simulink model "compassGaitSim_impacts"  (R2013a)
settings: Solver=ode45  StartTime=0.0  StopTime=20.0  FixedStep=0.01  MaxStep=0.02  MinStep=1e-8  RelTol=1e-3
values from neighbouring files (symbols this model uses):
  g = 9.81    [runSim.m]
  I1 = Is(1)    [PartialSolZeroDyn.m]    (also in impactDynamics_broken.m; runSim.m = 1)
  I2 = Is(2)    [PartialSolZeroDyn.m]    (also in impactDynamics_broken.m; runSim.m = 0.6)
  l1 = ls(1)    [PartialSolZeroDyn.m]    (also in impactDynamics_broken.m; runSim.m = 0.5)
  l2 = ls(2)    [PartialSolZeroDyn.m]    (also in impactDynamics_broken.m; runSim.m = 0.5)
  m1 = ms(1)    [PartialSolZeroDyn.m]    (also in impactDynamics_broken.m; runSim.m = 1.2)
  m2 = ms(2)    [PartialSolZeroDyn.m]    (also in impactDynamics_broken.m; runSim.m = 1.2)
  points = get(handles.uitable1, 'Data')'    [BezGui.m]    (also in BezGuiAttempt.m = [P0'; P1'; P2'; P3']; runSim.m = BezGuiAttempt')
undefined symbols (not defined in the file or in its folder): t1_0, t1d_0, t2_0, t2d_0
libraries: simulink x1
settings Model: CovHTMLOptions=-sRT=1 -aTS=1 -bRG=1 -bTC=1 -hTR=0 -nFC=0 -scm=1 -bcm=1 -xEv=0  Creator=yak  LastModifiedBy=yak

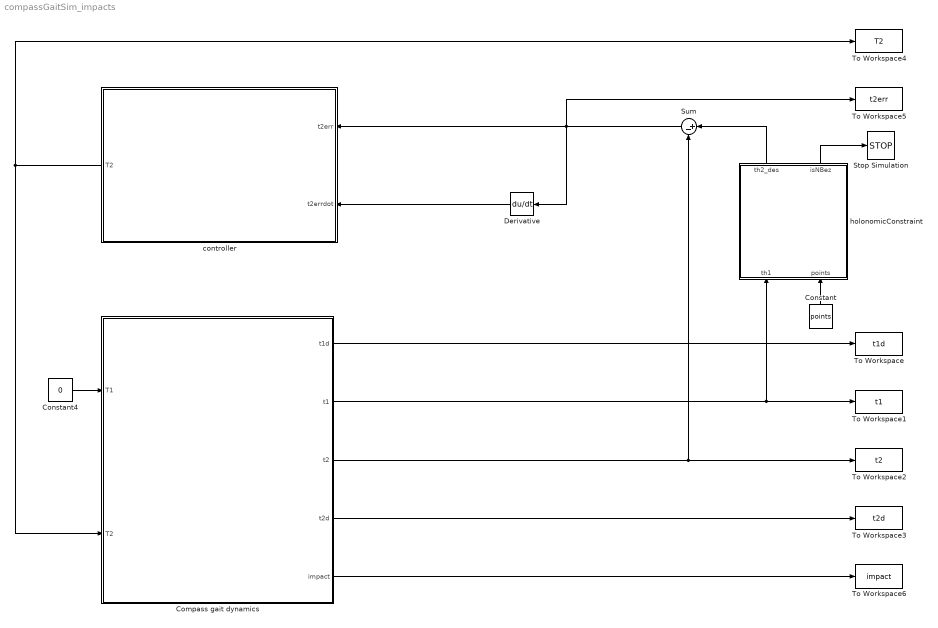
== system compassGaitSim_impacts ==
  Compass gait dynamics : Subsystem
  Constant : Constant  Value=points
  Constant4 : Constant  Value=0
  Derivative : Derivative
  Stop Simulation : Stop
  Sum : Sum  Inputs=|+-
  To Workspace : ToWorkspace  VariableName=t1d  SampleTime=-1  SaveFormat=Timeseries
  To Workspace1 : ToWorkspace  VariableName=t1  SampleTime=-1  SaveFormat=Timeseries
  To Workspace2 : ToWorkspace  VariableName=t2  SampleTime=-1  SaveFormat=Timeseries
  To Workspace3 : ToWorkspace  VariableName=t2d  SampleTime=-1  SaveFormat=Timeseries
  To Workspace4 : ToWorkspace  VariableName=T2  SampleTime=-1  SaveFormat=Timeseries
  To Workspace5 : ToWorkspace  VariableName=t2err  SampleTime=-1  SaveFormat=Timeseries
  To Workspace6 : ToWorkspace  VariableName=impact  SampleTime=-1  SaveFormat=Timeseries
  controller : MATLAB Function  TreatAsAtomicUnit=on
  holonomicConstraint : MATLAB Function  TreatAsAtomicUnit=on
  wires:
  controller/1(T2) -> Compass gait dynamics/2(T2), To Workspace4/1
  Compass gait dynamics/1(t1d) -> To Workspace/1
  Compass gait dynamics/2(t1) -> To Workspace1/1, holonomicConstraint/1(th1)
  Compass gait dynamics/3(t2) -> Sum/2, To Workspace2/1
  Compass gait dynamics/4(t2d) -> To Workspace3/1
  Constant4/1 -> Compass gait dynamics/1(T1)
  holonomicConstraint/1(th2_des) -> Sum/1
  Sum/1 -> To Workspace5/1, Derivative/1, controller/1(t2err)
  Derivative/1 -> controller/2(t2errdot)
  Constant/1 -> holonomicConstraint/2(points)
  holonomicConstraint/2(isNBez) -> Stop Simulation/1
  Compass gait dynamics/5(impact) -> To Workspace6/1

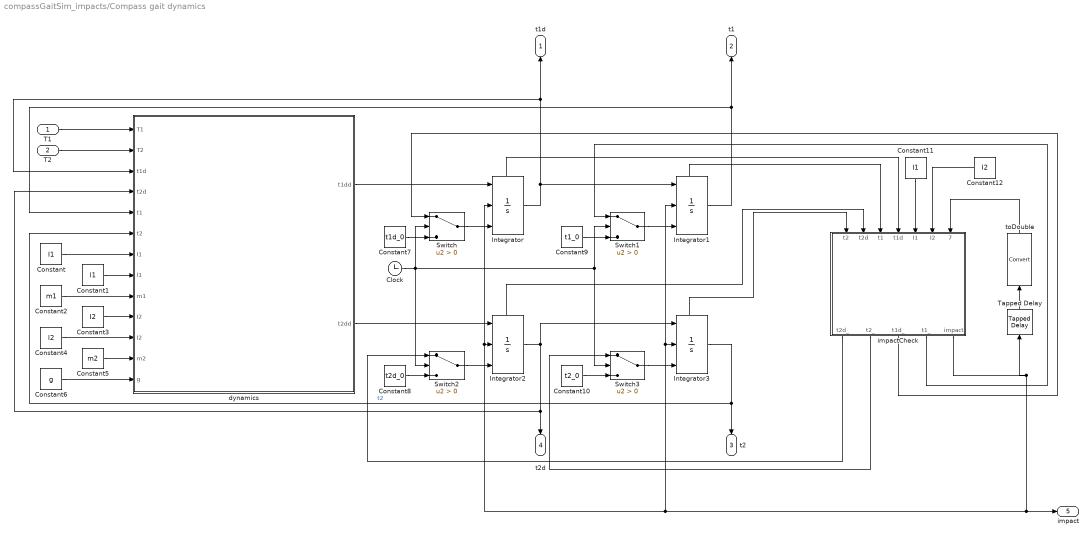
== system compassGaitSim_impacts/Compass gait dynamics ==
  T1 : Inport
  T2 : Inport  Port=2
  Clock : Clock
  Constant : Constant  Value=I1
  Constant1 : Constant  Value=l1
  Constant10 : Constant  Value=t2_0
  Constant11 : Constant  Value=I1
  Constant12 : Constant  Value=I2
  Constant2 : Constant  Value=m1
  Constant3 : Constant  Value=I2
  Constant4 : Constant  Value=l2
  Constant5 : Constant  Value=m2
  Constant6 : Constant  Value=g
  Constant7 : Constant  Value=t1d_0
  Constant8 : Constant  Value=t2d_0
  Constant9 : Constant  Value=t1_0
  Integrator{,1..3} (4 alike) : Integrator  ExternalReset=rising  InitialConditionSource=external  ShowStatePort=on
  Switch{,1..3} (4 alike) : Switch  Criteria=u2 > Threshold
  Tapped Delay : simulink/Discrete/Tapped Delay  vinit=1  samptime=-1  NumDelays=10  DelayOrder=Oldest  includeCurrent=off
  dynamics : MATLAB Function  TreatAsAtomicUnit=on
  impactCheck : MATLAB Function  TreatAsAtomicUnit=on
  toDouble : DataTypeConversion
  t1d : Outport
  t1 : Outport  Port=2
  t2 : Outport  Port=3
  t2d : Outport  Port=4
  impact : Outport  Port=5
  wires:
  T1/1 -> dynamics/1(T1)
  T2/1 -> dynamics/2(T2)
  dynamics/1(t1dd) -> Integrator/1
  Integrator/1 -> Integrator1/1, t1d/1, dynamics/3(t1d)
  Integrator2/1 -> Integrator3/1, t2d/1, dynamics/4(t2d)
  Integrator3/1 -> t2/1, dynamics/6(t2)  "t2"
  Integrator1/1 -> dynamics/5(t1), t1/1
  Constant2/1 -> dynamics/9(m1)
  Constant/1 -> dynamics/7(I1)
  Constant1/1 -> dynamics/8(l1)
  Constant3/1 -> dynamics/10(I2)
  Constant4/1 -> dynamics/11(l2)
  Constant5/1 -> dynamics/12(m2)
  Constant6/1 -> dynamics/13(g)
  Switch/1 -> Integrator/3
  Constant7/1 -> Switch/3
  Switch1/1 -> Integrator1/3
  Constant9/1 -> Switch1/3
  Switch2/1 -> Integrator2/3
  dynamics/2(t2dd) -> Integrator2/1
  Switch3/1 -> Integrator3/3
  Clock/1 -> Switch2/2, Switch3/2, Switch1/2, Switch/2
  Tapped Delay/1 -> toDouble/1
  impactCheck/5(impact) -> impact/1, Integrator1/2, Integrator3/2, Integrator/2, Integrator2/2, Tapped Delay/1
  toDouble/1 -> impactCheck/7(prev_impact)
  Integrator3/State -> impactCheck/1(t2)
  Integrator2/State -> impactCheck/2(t2d)
  Constant8/1 -> Switch2/3
  Constant10/1 -> Switch3/3
  impactCheck/1(t2d_) -> Switch2/1
  impactCheck/2(t2_) -> Switch3/1
  Integrator/State -> impactCheck/4(t1d)
  Integrator1/State -> impactCheck/3(t1)
  impactCheck/4(t1_) -> Switch1/1
  impactCheck/3(t1d_) -> Switch/1
  Constant11/1 -> impactCheck/5(I1)
  Constant12/1 -> impactCheck/6(I2)

== matlab function compassGaitSim_impacts/controller ==
  data: t2err input; t2errdot input; T2 output
function T2 = controller(t2err, t2errdot)
%#codegen

% Simple PD controller:
K_p = 1000;
K_d = 10;

t2err = mod(t2err, 2*pi);   % Ensure error is within 1 rotation

% Ensure error is in the range [-pi pi]
if t2err > pi
    t2err = -(2*pi - t2err);
elseif t2err < -pi
    t2err = 2*pi - t2err;
end

T2 = K_p*t2err + K_d*t2errdot;


end

== matlab function compassGaitSim_impacts/Compass gait dynamics/dynamics ==
  data: T1 input; t1dd output; T2 input; t1d input; t2d input; t1 input; t2 input; t2dd output; I1 input; l1 input; m1 input; I2 input; l2 input; m2 input; g input
function [t1dd, t2dd] = compassGaitDynamics(T1, T2, t1d, t2d, t1, t2, ...
    I1, l1, m1, I2, l2, m2, g)
%#codegen

c1 = cos(t1);
c2 = cos(t2);
s2 = sin(t2);
c12 = cos(t1 + t2);


% Equations in terms of T1 and T2 are derived, then the solution in terms
% of the angle accelerations have been pre-solved. The output is below.
t1dd = (4*I2*T1 - 4*I2*T2 + T1*l2^2*m2 - T2*l2^2*m2 - ...
    c1*g*l1*l2^2*m2^2 - 2*I2*c1*g*l1*m1 - 4*I2*c1*g*l1*m2 - ...
    2*T2*c2*l1*l2*m2 + (l1*l2^3*m2^2*s2*t1d^2)/2 + ...
    (l1*l2^3*m2^2*s2*t2d^2)/2 + 2*I2*l1*l2*m2*s2*t1d^2 + ...
    2*I2*l1*l2*m2*s2*t2d^2 - (c1*g*l1*l2^2*m1*m2)/2 + ...
    c2*l1^2*l2^2*m2^2*s2*t1d^2 + c2*c12*g*l1*l2^2*m2^2 + ...
    l1*l2^3*m2^2*s2*t1d*t2d + 4*I2*l1*l2*m2*s2*t1d*t2d)/ ...
    (- c2^2*l1^2*l2^2*m2^2 + l1^2*l2^2*m2^2 + ...
    4*I2*l1^2*m2 + I1*l2^2*m2 + 4*I1*I2);

t2dd = -(4*I2*T1 - 4*I1*T2 - 4*I2*T2 + T1*l2^2*m2 - 4*T2*l1^2*m2 - ...
    T2*l2^2*m2 - c1*g*l1*l2^2*m2^2 + 2*c12*g*l1^2*l2*m2^2 - ...
    2*I2*c1*g*l1*m1 - 4*I2*c1*g*l1*m2 + 2*I1*c12*g*l2*m2 + ...
    2*T1*c2*l1*l2*m2 - 4*T2*c2*l1*l2*m2 + (l1*l2^3*m2^2*s2*t1d^2)/2 + ...
    2*l1^3*l2*m2^2*s2*t1d^2 + (l1*l2^3*m2^2*s2*t2d^2)/2 + ...
    2*I1*l1*l2*m2*s2*t1d^2 + 2*I2*l1*l2*m2*s2*t1d^2 + ...
    2*I2*l1*l2*m2*s2*t2d^2 - (c1*g*l1*l2^2*m1*m2)/2 + ...
    2*c2*l1^2*l2^2*m2^2*s2*t1d^2 + c2*l1^2*l2^2*m2^2*s2*t2d^2 - ...
    2*c1*c2*g*l1^2*l2*m2^2 + c2*c12*g*l1*l2^2*m2^2 + ...
    l1*l2^3*m2^2*s2*t1d*t2d + 4*I2*l1*l2*m2*s2*t1d*t2d + ...
    2*c2*l1^2*l2^2*m2^2*s2*t1d*t2d - c1*c2*g*l1^2*l2*m1*m2)/(- ...
    c2^2*l1^2*l2^2*m2^2 + l1^2*l2^2*m2^2 + 4*I2*l1^2*m2 + I1*l2^2*m2 + ...
    4*I1*I2);

end

== matlab function compassGaitSim_impacts/holonomicConstraint ==
  data: th1 input; points input; th2_des output; isNBez output
function [th2_des, isNBez] = holonomicConstraint(th1, points)
%#codegen

coder.extrinsic('holonomic');
th2_des = zeros(1,1,'double');
isNBez = false;

% Use constraint as defined by function in holonomic.m
th2_des = holonomic(th1, points);

end

== matlab function compassGaitSim_impacts/Compass gait dynamics/impactCheck ==
  data: t2d_ output; t2_ output; t1d_ output; t1_ output; t2 input; t2d input; t1 input; t1d input; I1 input; I2 input; impact output; prev_impact input
function [t2d_, t2_, t1d_, t1_, impact] = impact(t2, t2d, ...
    t1, t1d, I1, I2, prev_impact)
%#codegen

HORIZ_THRESH = 0.03;
EXCEPTION_THRESH = 0.1;
delta = zeros(1,1,'double');

isOnHoriz = abs(t2 + 2*t1) < HORIZ_THRESH; % Cond: t2 = -2*t1
% Contract the swing leg in the first half of the swing to avoid impact
isShorter = t2 + pi < EXCEPTION_THRESH; % t2 < -pi for first half of swing

% Check for impact condition
if isOnHoriz && ~isShorter && min(~prev_impact)
    t1_ = pi - t1;
    t2_ = -2*pi - t2;
    % Conservation of momentum + invariance of zero dynamics
    delta = ( t1d*(I1+I2) + t2d*I2 )/( t1d*(I1+2*I2) + t2d*(I1+I2) );
    t1d = delta*t1d;
    t2d = delta*t2d;
    % Change of coordinates
    t1d_ = t1d + t2d;
    t2d_ = t2d;
    impact = true;
else
    t1_ = t1;
    t2_ = t2;
    t1d_ = t1d;
    t2d_ = t2d;
    impact = false;
end

end
